simulink model "exp5_3"  (Simulink 3.00)
settings: Solver=ode45  SolverMode=SingleTasking  StartTime=0.0  StopTime=2  RelTol=1e-3  AbsTol=1e-6
settings Model: RTWTemplateMakefile=grt_vc.tmf

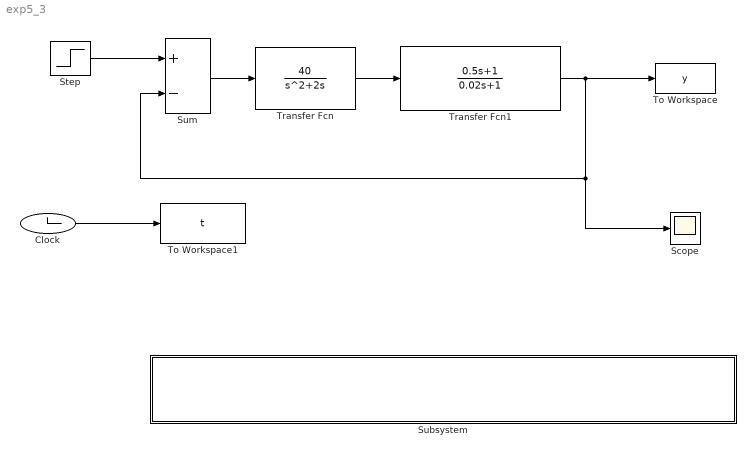
== system exp5_3 ==
  Clock : Clock
      settings: DisplayTime=off  Decimation=10
  Scope : Scope
      settings: TimeRange=2  YMin=0  YMax=1.4  SaveToWorkspace=off  SaveName=ScopeData
  Step : Step  Time=0  Before=0  After=1  SampleTime=0
  Subsystem : Subsystem
      settings: OpenFcn=ploty
      mask Display: disp('After simulation Double Click Here to Plot The Result')
  Sum : Sum  Inputs=+-  SaturateOnIntegerOverflow=on
  To Workspace : ToWorkspace  VariableName=y  SampleTime=-1  SaveFormat=Matrix
  To Workspace1 : ToWorkspace  VariableName=t  SampleTime=-1  SaveFormat=Matrix
  Transfer Fcn : TransferFcn  Numerator=[40]  Denominator=[1 2 0]
  Transfer Fcn1 : TransferFcn  Numerator=[0.5 1]  Denominator=[0.02 1]
  wires:
  Transfer Fcn1/1 -> To Workspace/1, Sum/2, Scope/1
  Transfer Fcn/1 -> Transfer Fcn1/1
  Sum/1 -> Transfer Fcn/1
  Step/1 -> Sum/1
  Clock/1 -> To Workspace1/1

== system exp5_3/Subsystem ==
